simulink library "ece3413"  (R2018b)
settings: Solver=VariableStepAuto  StartTime=0.0  StopTime=10.0  RelTol=1e-3
settings Model: Creator=lbai  LastModifiedBy=Adam0

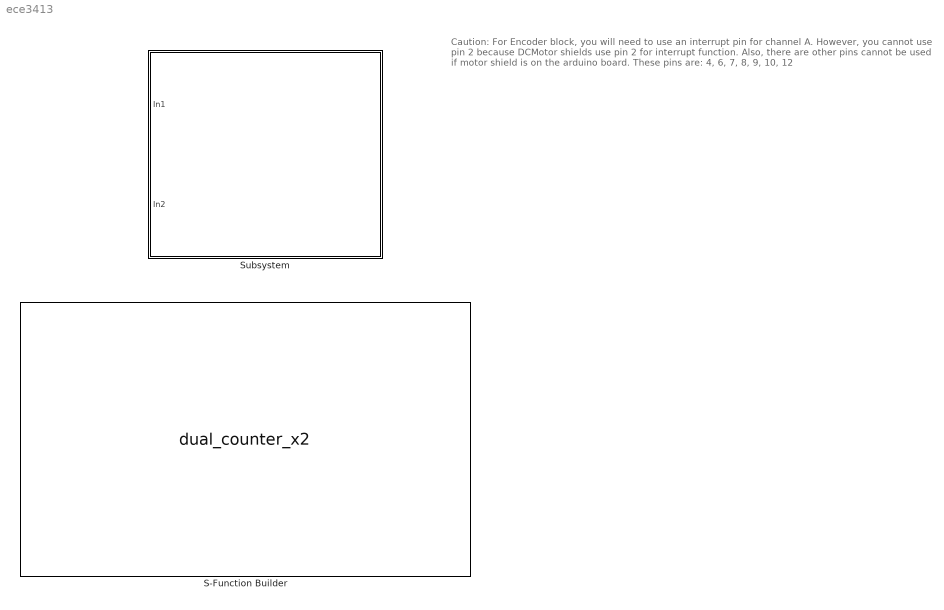
== system ece3413 ==
  note: Caution: For Encoder block, you will need to use an interrupt pin for channel A. However, you cannot use pin 2 because DCMotor shields use pin 2 for interrupt function. Also, there are other pins cannot be used if motor shield is on the arduino board. These pins are: 4, 6, 7, 8, 9, 10, 12
  S-Function Builder : S-Function  InitFcn=try, set_param(gcb,'FunctionName','dual_counter_x2'), end  FunctionName=dual_counter_x2  SFunctionModules=dual_counter_x2_wrapper  SFunctionDeploymentMode=off  EnableBusSupport=off  mask(S-Function Builder){}
      mask help: Simulink:masks:SFunctionBuilder_MD
      mask init:
      | val = [[.9  0.75 0.75 1 1 .9 .9 1]',[1 1 0.75 0.75 .9 .9 1 .9]'];try , sys = get_param(gcb,'SfunBuilderFcnName');if isempty(sys), sys = get_param(gcb,'FunctionName'); end,catch, sys = get_param(gcb,'FunctionName'); end
      settings: CopyFcn=set_param(gcbh,'LinkStatus','none')  PreSaveFcn=try, set_param(gcb,'FunctionName','dual_counter_x2'), end  OpenFcn=sfunctionwizard(gcbh)
      mask Display: plot(val(:,1),val(:,2)),disp(sys), port_label('input',1,'encoder1a'), port_label('input',2,'encoder1b'), port_label('input',3,'encoder2a'), port_label('input',4,'encoder2b'), port_label('output',1,'count1'), port_label('output',2,'count2')
  Subsystem : Subsystem
      mask Display:
      | image('motor.jpg');
      | port_label('input', 1, 'motor#')
      | port_label('input', 2, 'speed')
      | port_label('output', 1, 'current')

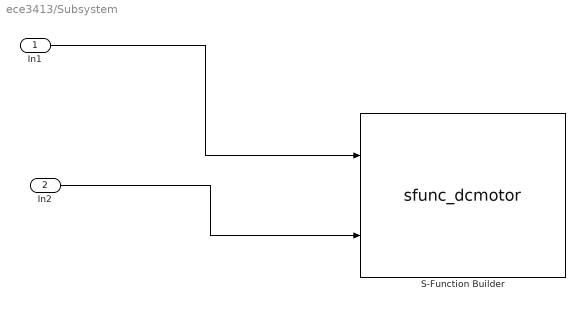
== system ece3413/Subsystem ==
  In1 : Inport
  In2 : Inport  Port=2
  S-Function Builder : S-Function  InitFcn=try, set_param(gcb,'FunctionName','sfunc_dcmotor'), end  FunctionName=sfunc_dcmotor  SFunctionModules=sfunc_dcmotor_wrapper  SFunctionDeploymentMode=off  EnableBusSupport=off  mask(S-Function Builder){}
      mask help: Simulink:masks:SFunctionBuilder_MD
      mask init: same as ece3413/S-Function Builder
      settings: CopyFcn=set_param(gcbh,'LinkStatus','none')  PreSaveFcn=try, set_param(gcb,'FunctionName','sfunc_dcmotor'), end  OpenFcn=sfunctionwizard(gcbh)
      mask Display: plot(val(:,1),val(:,2)),disp(sys), port_label('input',1,'spd1'), port_label('input',2,'spd2')
  wires:
  In2/1 -> S-Function Builder/2
  In1/1 -> S-Function Builder/1
